simulink model "LEGO_HW"  (R2023a)
settings: Solver=ode3  StartTime=0.0  StopTime=inf  FixedStep=Ts  RelTol=1e-3
InitFcn:
  | lego_drive_openloop_InitData.mdl = get_param(bdroot,'Name');
  | lego_drive_openloop_InitData.cs = getActiveConfigSet(lego_drive_openloop_InitData.mdl);
values from neighbouring files (symbols this model uses):
  a_gc = 0.8    [run_LEGO_HW.m]
  a_gd = 0.999    [run_LEGO_HW.m]
  dot_phi_ref = -1.8    [run_LEGO_HW.m]
  dot_theta_ref = 7    [run_LEGO_HW.m]
  KDtheta = Kpp(3)    [run_LEGO_HW.m]
  KIpsi = Kpp(2)    [run_LEGO_HW.m]
  KItheta = Kpp(5)    [run_LEGO_HW.m]
  Kopenloop = -A2(2,2)/B2(2,1)    [run_LEGO_HW.m]
  KPphi = -6    [run_LEGO_HW.m]
  KPpsi = Kpp(4)    [run_LEGO_HW.m]
  KPtheta = Kpp(1)    [run_LEGO_HW.m]
  maxacc = 2    [run_LEGO_HW.m]
  R = 0.027    [run_LEGO_HW.m]
  thetamy = 2.8    [run_LEGO_HW.m]
  thres_yaw = -1    [run_LEGO_HW.m]
  Ts = 0.004    [run_LEGO_HW.m]
  W = 0.14    [run_LEGO_HW.m]
undefined symbols (not defined in the file or in its folder): DiscIntNeverNeededParam
libraries: legoev3lib x8, simulink x4, simulink_extras x3, shared_linuxserviceslib x1, simulink_need_slupdate x1
PreSaveFcn:
  | set_param(gcs, 'Location',[35 56 895 605])
CloseFcn:
  | clear lego_drive_openloop_InitData
settings Model: SimulationMode=external  ExtModeTrigDuration=2  Creator=The MathWorks, Inc.  LastModifiedBy=lab5
settings SolverCC: AlgebraicLoopSolver=TrustRegion  PositivePriorityOrder=on
settings DataIOCC: LimitDataPoints=on  SaveFormat=Array  SaveOutput=off  SignalLogging=off  DSMLogging=off  SaveTime=off  ReturnWorkspaceOutputs=off
settings OptimizationCC: ExpressionDepthLimit=2147483647  LifeSpan=Inf  MaxStackSize=64
settings DebuggingCC: UnderspecifiedInitializationDetection=Classic  MergeDetectMultiDrivingBlocksExec=none  InheritedTsInSrcMsg=none  ParameterPrecisionLossMsg=none  FcnCallInpInsideContextMsg=warning  UnconnectedInputMsg=warning  UnconnectedOutputMsg=warning  UnconnectedLineMsg=warning  AllowSymbolicDim=off  StateNameClashWarn=warning  SFUnexpectedBacktrackingDiag=warning  SFNoUnconditionalDefaultTransitionDiag=warning  SFExecutionAtInitializationDiag=none  ArithmeticOperatorsInVariantConditions=warning
settings HardwareCC: ProdBitPerPointer=32  ProdBitPerSizeT=32  ProdBitPerPtrDiffT=32  ProdLargestAtomicInteger=Long  ProdWordSize=32  ProdHWDeviceType=ARM Compatible->ARM 9  UseEmbeddedCoderFeatures=off  UseSimulinkCoderFeatures=off
settings ModelReferenceCC: UpdateModelReferenceTargets=Force  EnableRefExpFcnMdlSchedulingChecks=on  PropagateSignalLabelsOutOfModel=off
settings SFSimCC: SimUseLocalCustomCode=off  CustomCodeUndefinedFunction=UseInterfaceOnly
settings RTWCC: Description=Embedded Coder  SystemTargetFile=ert.tlc  HardwareBoard=LEGO MINDSTORMS EV3  TemplateMakefile=ert_default_tmf  GenerateReport=on  RTWVerbose=off  RTWUseLocalCustomCode=off  Toolchain=Sourcery G++ Lite v2009q3  LaunchReport=on  DLArmComputeVersion=19.05
settings CodeAppCC: ForceParamTrailComments=on  OperatorAnnotations=on  StateflowObjectComments=on  MATLABSourceComments=on
settings ERTTargetCC: MultiwordLength=2048  ERTCustomFileBanners=off  SupportContinuousTime=on  SupportNonInlinedSFcns=on  RemoveResetFunc=off  ModelStepFunctionPrototypeControlCompliant=off
settings ConfigComp: CovMetricSettings=dw  CovSaveCumulativeToWorkspaceVar=on  CovSaveSingleToWorkspaceVar=on  CovExternalEMLEnable=off  CovSFcnEnable=off

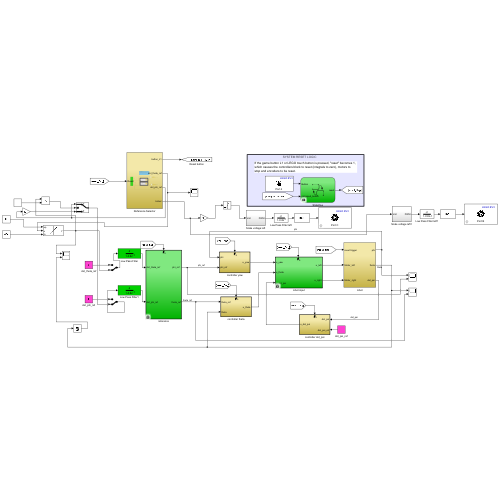
[thumbnail: Simulink's stored preview of the top-level diagram]
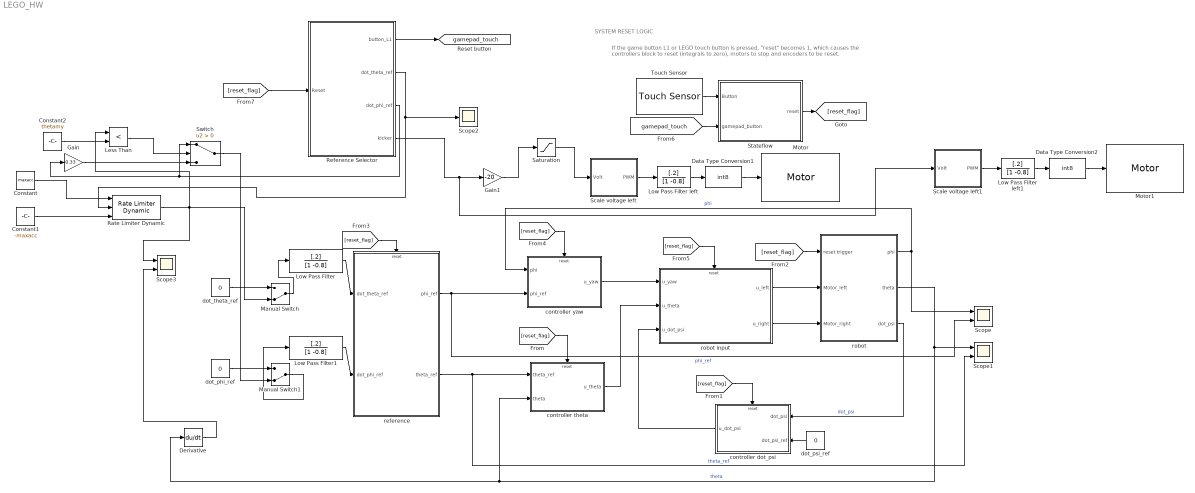
== system LEGO_HW ==
  note: If the game button L1 or LEGO touch button is pressed, "reset" becomes 1, which causes the controllers block to reset (integrals to zero), motors to stop and encoders to be reset.
  note: SYSTEM RESET LOGIC
  Constant : Constant  Value=maxacc
  Constant1 : Constant  Value=-maxacc
  Constant2 : Constant  Value=thetamy
  Data Type Conversion1 : DataTypeConversion  OutDataTypeStr=int8  SaturateOnIntegerOverflow=off  RndMeth=Floor
  Data Type Conversion2 : DataTypeConversion  OutDataTypeStr=int8  SaturateOnIntegerOverflow=off  RndMeth=Floor
  Derivative : Derivative
  Gain : Gain  Gain=0.33
  Gain1 : Gain  Gain=-20
  Less Than : RelationalOperator  Operator=<  OutDataTypeStr=boolean  RndMeth=Simplest  InputSameDT=off
  Low Pass Filter : DiscreteFilter  Numerator=[.2]  Denominator=[1 -0.8]  SampleTime=Ts
  Low Pass Filter left : DiscreteFilter  Numerator=[.2]  Denominator=[1 -0.8]
  Low Pass Filter left1 : DiscreteFilter  Numerator=[.2]  Denominator=[1 -0.8]
  Low Pass Filter1 : DiscreteFilter  Numerator=[.2]  Denominator=[1 -0.8]  SampleTime=Ts
  Manual Switch : ManualSwitch  CurrentSetting=0
  Manual Switch1 : ManualSwitch  CurrentSetting=0
  Motor : legoev3lib/Motor  sportNumber=C  sstopAction=Brake
  Motor1 : legoev3lib/Motor  sportNumber=B  sstopAction=Brake
  Rate Limiter Dynamic : simulink/Discontinuities/Rate Limiter Dynamic
  Reference Selector : Subsystem
  Saturation : Saturate  UpperLimit=2  LowerLimit=-20
  Scale voltage left : Subsystem
  Scale voltage left1 : Subsystem
  Scope : Scope  NumInputPorts=2
  Scope1 : Scope  NumInputPorts=2
  Scope2 : Scope
  Scope3 : Scope  NumInputPorts=2
  Stateflow : Stateflow chart  TreatAsAtomicUnit=on  SystemSampleTime=Ts
      settings: CopyFcn=|
      | % delete the link so that this is editable
      | set_param(gcb, 'LinkStatus', 'none');
  Switch : Switch  Criteria=u2 > Threshold  SaturateOnIntegerOverflow=off  InputSameDT=off
  Touch Sensor : legoev3lib/Touch Sensor  portNumber=4  sampleTime=Ts
  controller dot_psi : Subsystem
  controller theta : Subsystem
  controller yaw : Subsystem
  dot_phi_ref : Constant  Value=0
  dot_psi_ref : Constant  Value=0  VectorParams1D=off
  dot_theta_ref : Constant  Value=0
  reference : Subsystem
  robot : Subsystem  VariantControl=DoSim
  robot input : Subsystem
  tag scope: gamepad_touch=global
  wires:
  controller yaw/1(u_yaw) -> robot input/1(u_yaw)
  controller theta/1(u_theta) -> robot input/2(u_theta)
  controller dot_psi/1(u_dot_psi) -> robot input/3(u_dot_psi)
  reference/1("phi_ref  ") -> Scope/2, controller yaw/2(phi_ref)  "phi_ref"
  reference/2(theta_ref) -> Scope1/2, controller theta/1(theta_ref)  "theta_ref"
  dot_psi_ref/1 -> controller dot_psi/2(dot_psi_ref)
  robot/3(dot_psi) -> controller dot_psi/1(dot_psi)  "dot_psi"
  robot/2(theta) -> Derivative/1, controller theta/2(theta), Scope1/1  "theta"
  robot input/1(u_left) -> robot/2(Motor_left)
  robot input/2(u_right) -> robot/3(Motor_right)
  Stateflow/1(reset) -> [reset_flag]
  [reset_flag] -> controller theta/Reset
  [reset_flag] -> controller dot_psi/Reset
  [reset_flag] -> robot/1(reset trigger)
  [reset_flag] -> controller yaw/Reset
  [reset_flag] -> reference/Reset
  [reset_flag] -> robot input/Reset
  Touch Sensor/1 -> Stateflow/1(Button)
  robot/1(phi) -> controller yaw/1(phi), Scope/1  "phi"
  dot_theta_ref/1 -> Manual Switch/1
  dot_phi_ref/1 -> Manual Switch1/1
  [gamepad_touch] -> Stateflow/2(gamepad_button)
  Reference Selector/2(dot_theta_ref) -> Rate Limiter Dynamic/2, Scope2/1
  Reference Selector/4(kicker) -> Scale voltage left1/1(Volt), Gain1/1
  Reference Selector/1(button_L1) -> [gamepad_touch]
  [reset_flag] -> Reference Selector/1(Reset)
  Manual Switch/1 -> Low Pass Filter/1
  Low Pass Filter/1 -> reference/1(dot_theta_ref)
  Low Pass Filter1/1 -> reference/2(dot_phi_ref)
  Manual Switch1/1 -> Low Pass Filter1/1
  Constant/1 -> Rate Limiter Dynamic/1
  Constant1/1 -> Rate Limiter Dynamic/3
  Rate Limiter Dynamic/1 -> Less Than/1, Scope3/1, Manual Switch/2
  Derivative/1 -> Scope3/2
  Reference Selector/3(dot_phi_ref) -> Gain/1, Switch/1
  Switch/1 -> Manual Switch1/2
  Constant2/1 -> Less Than/2
  Less Than/1 -> Switch/2
  Gain/1 -> Switch/3
  Scale voltage left/1(PWM) -> Low Pass Filter left/1
  Low Pass Filter left/1 -> Data Type Conversion1/1
  Data Type Conversion1/1 -> Motor/1
  Gain1/1 -> Saturation/1
  Saturation/1 -> Scale voltage left/1(Volt)
  Scale voltage left1/1(PWM) -> Low Pass Filter left1/1
  Low Pass Filter left1/1 -> Data Type Conversion2/1
  Data Type Conversion2/1 -> Motor1/1

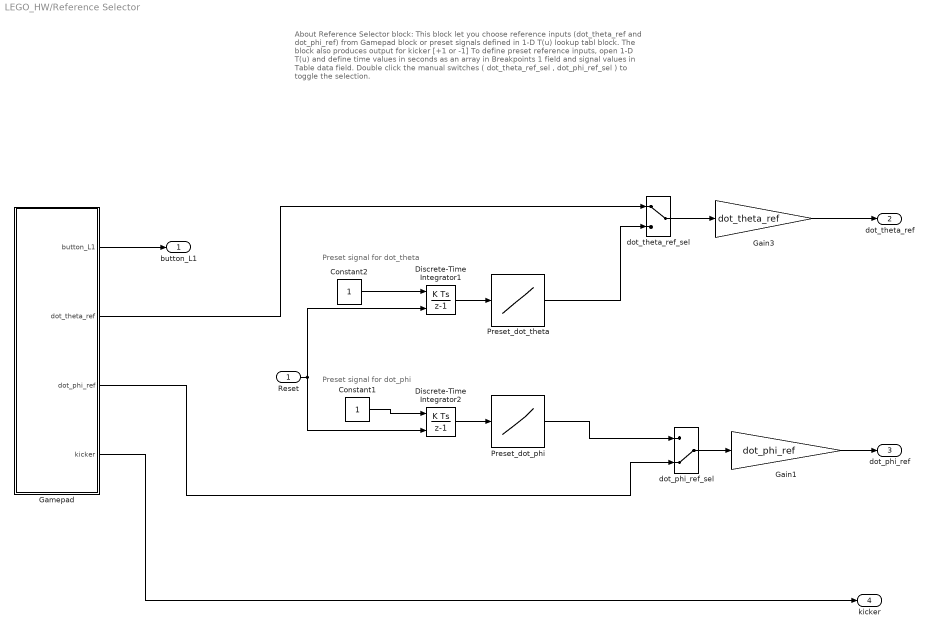
== system LEGO_HW/Reference Selector ==
  note: Preset signal for dot_theta
  note: About Reference Selector block:
      | This block let you choose reference inputs (dot_theta_ref and dot_phi_ref) from Gamepad block or preset signals defined in 1-D T(u) lookup tabl block. The block also produces output for kicker [+1 or -1]
      |
      | To define preset reference inputs, open 1-D T(u) and define time values in seconds as an array in Breakpoints 1 field and signal values in Table data field.
      |
      | Double click the manual switches ( dot_theta_ref_sel , dot_phi_ref_sel ) to toggle the selection.
  note: Preset signal for dot_phi
  Reset : Inport
  Constant1 : Constant
  Constant2 : Constant
  Discrete-Time Integrator1 : DiscreteIntegrator  ExternalReset=level  SampleTime=Ts  ICPrevOutput=DiscIntNeverNeededParam  ICPrevScaledInput=DiscIntNeverNeededParam
  Discrete-Time Integrator2 : DiscreteIntegrator  ExternalReset=level  SampleTime=Ts  ICPrevOutput=DiscIntNeverNeededParam  ICPrevScaledInput=DiscIntNeverNeededParam
  Gain1 : Gain  Gain=dot_phi_ref
  Gain3 : Gain  Gain=dot_theta_ref
  Gamepad : Subsystem
  Preset_dot_phi : Lookup_n-D  NumberOfTableDimensions=1  BreakpointsForDimension1=[0 1 2 3 4 5 6 9.1 10.8 11 12 12.1 12.2 13 14 15 16 17 18 19 20]  Table=[0;0;0;0;0;0;0;8;0;0;0;0;0;0;0;0;0;0;0;0;0]  InterpMethod=Flat  InternalRulePriority=Speed  RndMeth=Ceiling
  Preset_dot_theta : Lookup_n-D  NumberOfTableDimensions=1  BreakpointsForDimension1=[0;1;2;2.5;2.6;2.7;3.7;4.8;5.9;7;8;9;10;11;11.5;12.4;13;14;15;16;17;18;19;20;21;22]  Table=[0;0;0;0;0;0;0.5;1.5;2.5;2.7;2.5;1;0;0;0.5;1.3;2;2.3;2.5;2.1;1.5;0.5;0;0;0;0]  InterpMethod=Cubic spline  InternalRulePriority=Speed  RndMeth=Ceiling
  dot_phi_ref_sel : ManualSwitch  CurrentSetting=0
  dot_theta_ref_sel : ManualSwitch
  button_L1 : Outport
  dot_theta_ref : Outport  Port=2
  dot_phi_ref : Outport  Port=3
  kicker : Outport  Port=4
  wires:
  Discrete-Time Integrator1/1 -> Preset_dot_theta/1
  Gamepad/1(button_L1) -> button_L1/1
  Gamepad/2(dot_theta_ref) -> dot_theta_ref_sel/1
  Preset_dot_theta/1 -> dot_theta_ref_sel/2
  Gamepad/4(kicker) -> kicker/1
  dot_theta_ref_sel/1 -> Gain3/1
  dot_phi_ref_sel/1 -> Gain1/1
  Gain3/1 -> dot_theta_ref/1
  Discrete-Time Integrator2/1 -> Preset_dot_phi/1
  Reset/1 -> Discrete-Time Integrator2/2, Discrete-Time Integrator1/2
  Preset_dot_phi/1 -> dot_phi_ref_sel/1
  Gamepad/3(dot_phi_ref) -> dot_phi_ref_sel/2
  Gain1/1 -> dot_phi_ref/1
  Constant2/1 -> Discrete-Time Integrator1/1
  Constant1/1 -> Discrete-Time Integrator2/1

== system LEGO_HW/Scale voltage left ==
  Volt : Inport
  PWM --> Volts (for V_batt = 8000mV) : Gain  Gain=100/8.087
  Saturation : Saturate  UpperLimit=100  LowerLimit=-100
  PWM : Outport  VectorParamsAs1DForOutWhenUnconnected=off
  wires:
  PWM --> Volts (for V_batt = 8000mV)/1 -> Saturation/1
  Volt/1 -> PWM --> Volts (for V_batt = 8000mV)/1
  Saturation/1 -> PWM/1

== system LEGO_HW/Scale voltage left1 ==
  Volt : Inport
  PWM --> Volts (for V_batt = 8000mV) : Gain  Gain=100/8.087
  Saturation : Saturate  UpperLimit=100  LowerLimit=-100
  PWM : Outport  VectorParamsAs1DForOutWhenUnconnected=off
  wires:
  PWM --> Volts (for V_batt = 8000mV)/1 -> Saturation/1
  Volt/1 -> PWM --> Volts (for V_batt = 8000mV)/1
  Saturation/1 -> PWM/1

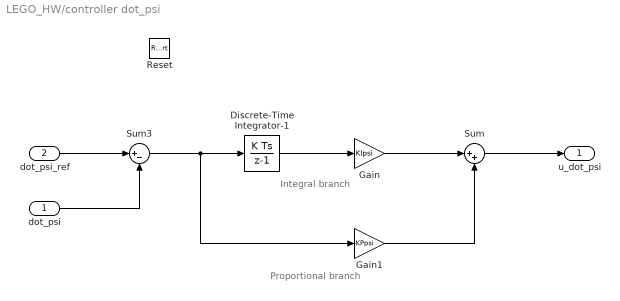
== system LEGO_HW/controller dot_psi ==
  note: Proportional branch
  note: Integral branch
  dot_psi : Inport
  dot_psi_ref : Inport  Port=2
  Reset : ResetPort  DisableCoverage=on
  Discrete-Time Integrator-1 : DiscreteIntegrator  SampleTime=Ts  ICPrevOutput=DiscIntNeverNeededParam  ICPrevScaledInput=DiscIntNeverNeededParam
  Gain : Gain  Gain=KIpsi
  Gain1 : Gain  Gain=KPpsi
  Sum : Sum  Inputs=|++  OutDataTypeStr=Inherit: Same as first input
  Sum3 : Sum  Inputs=|+-  OutDataTypeStr=Inherit: Same as first input
  u_dot_psi : Outport  VectorParamsAs1DForOutWhenUnconnected=off
  wires:
  dot_psi/1 -> Sum3/2
  dot_psi_ref/1 -> Sum3/1
  Discrete-Time Integrator-1/1 -> Gain/1
  Sum3/1 -> Gain1/1, Discrete-Time Integrator-1/1
  Sum/1 -> u_dot_psi/1
  Gain1/1 -> Sum/2
  Gain/1 -> Sum/1

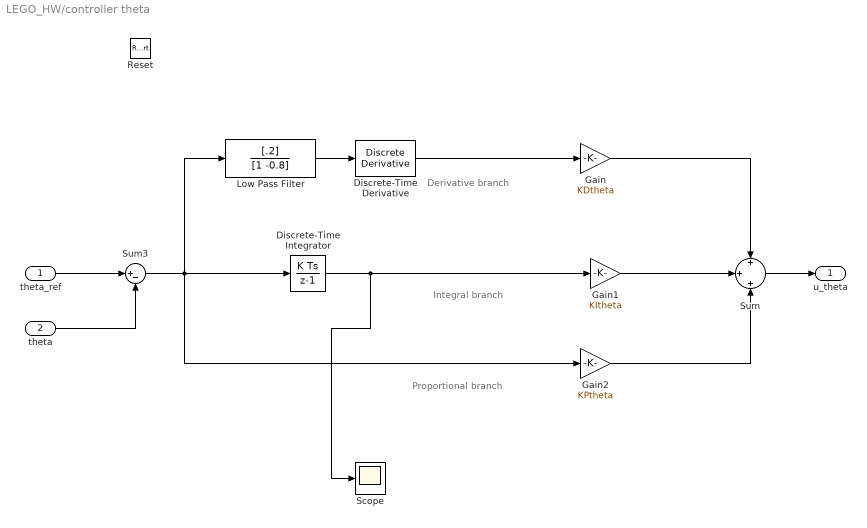
== system LEGO_HW/controller theta ==
  note: Proportional branch
  note: Integral branch
  note: Derivative branch
  theta_ref : Inport
  theta : Inport  Port=2
  Reset : ResetPort  DisableCoverage=on
  Discrete-Time Derivative : simulink/Discrete/Discrete Derivative  gainval=1.0  ICPrevScaledInput=0.0  OutMin=[]  OutMax=[]  OutDataType=fixdt(1, 16)  OutScaling=2^-10  DoSatur=off
  Discrete-Time Integrator : DiscreteIntegrator  SampleTime=Ts  ICPrevOutput=DiscIntNeverNeededParam  ICPrevScaledInput=DiscIntNeverNeededParam
  Gain : Gain  Gain=KDtheta
  Gain1 : Gain  Gain=KItheta
  Gain2 : Gain  Gain=KPtheta
  Low Pass Filter : DiscreteFilter  Numerator=[.2]  Denominator=[1 -0.8]  SampleTime=Ts
  Scope : Scope
  Sum : Sum  Inputs=+|+|+  OutDataTypeStr=Inherit: Same as first input
  Sum3 : Sum  Inputs=|+-  OutDataTypeStr=Inherit: Same as first input
  u_theta : Outport  VectorParamsAs1DForOutWhenUnconnected=off
  wires:
  theta/1 -> Sum3/2
  theta_ref/1 -> Sum3/1
  Discrete-Time Integrator/1 -> Scope/1, Gain1/1
  Discrete-Time Derivative/1 -> Gain/1
  Sum3/1 -> Gain2/1, Discrete-Time Integrator/1, Low Pass Filter/1
  Sum/1 -> u_theta/1
  Gain2/1 -> Sum/3
  Gain1/1 -> Sum/2
  Gain/1 -> Sum/1
  Low Pass Filter/1 -> Discrete-Time Derivative/1

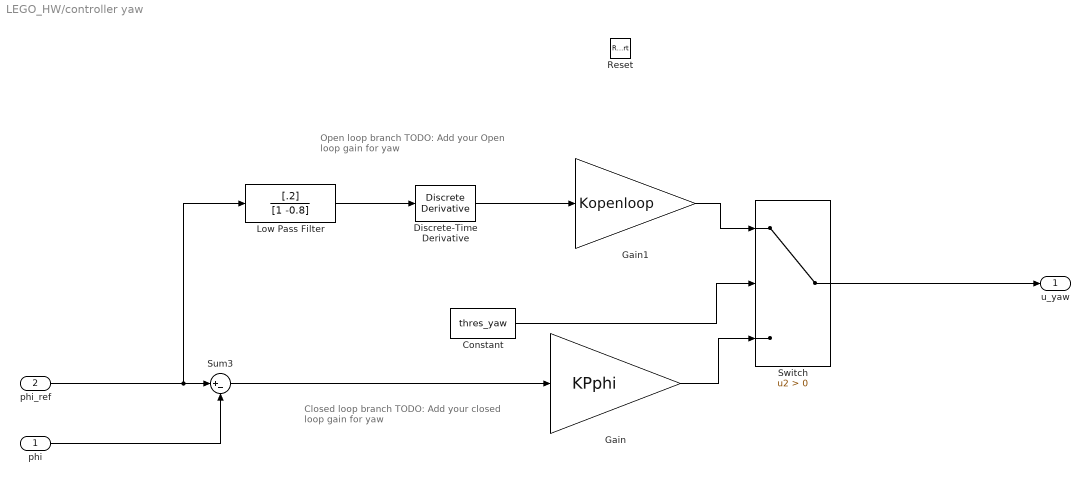
== system LEGO_HW/controller yaw ==
  note: Closed loop branch
      | TODO: Add your closed loop gain for yaw
  note: Open loop branch
      | TODO: Add your Open loop gain for yaw
  phi : Inport
  phi_ref : Inport  Port=2
  Reset : ResetPort  DisableCoverage=on
  Constant : Constant  Value=thres_yaw
  Discrete-Time Derivative : simulink/Discrete/Discrete Derivative  gainval=1.0  ICPrevScaledInput=0.0  OutMin=[]  OutMax=[]  OutDataType=fixdt(1, 16)  OutScaling=2^-10  DoSatur=off
  Gain : Gain  Gain=KPphi
  Gain1 : Gain  Gain=Kopenloop
  Low Pass Filter : DiscreteFilter  Numerator=[.2]  Denominator=[1 -0.8]  SampleTime=Ts
  Sum3 : Sum  Inputs=|+-
  Switch : Switch  Criteria=u2 > Threshold  SaturateOnIntegerOverflow=off  InputSameDT=off
  u_yaw : Outport  VectorParamsAs1DForOutWhenUnconnected=off
  wires:
  phi/1 -> Sum3/2
  phi_ref/1 -> Low Pass Filter/1, Sum3/1
  Sum3/1 -> Gain/1
  Discrete-Time Derivative/1 -> Gain1/1
  Constant/1 -> Switch/2
  Low Pass Filter/1 -> Discrete-Time Derivative/1
  Gain1/1 -> Switch/1
  Switch/1 -> u_yaw/1
  Gain/1 -> Switch/3

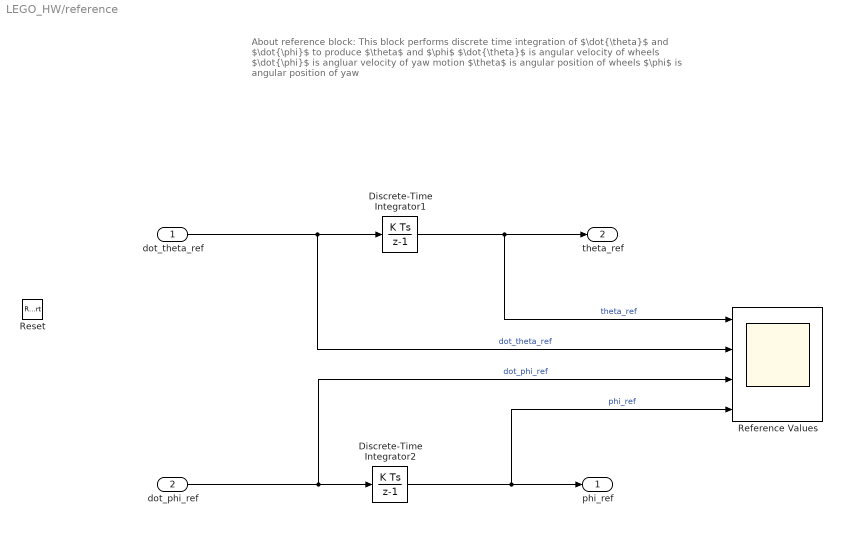
== system LEGO_HW/reference ==
  note: About reference block:
      | This block performs discrete time integration of $\dot{\theta}$ and $\dot{\phi}$ to produce $\theta$ and $\phi$
      | $\dot{\theta}$ is angular velocity of wheels
      | $\dot{\phi}$ is angluar velocity of yaw motion
      | $\theta$ is angular position of wheels
      | $\phi$ is angular position of yaw
  dot_theta_ref : Inport
  dot_phi_ref : Inport  Port=2
  Reset : ResetPort  DisableCoverage=on
  Discrete-Time Integrator1 : DiscreteIntegrator  SampleTime=Ts  ICPrevOutput=DiscIntNeverNeededParam  ICPrevScaledInput=DiscIntNeverNeededParam
  Discrete-Time Integrator2 : DiscreteIntegrator  SampleTime=Ts  ICPrevOutput=DiscIntNeverNeededParam  ICPrevScaledInput=DiscIntNeverNeededParam
  Reference Values : Scope  NumInputPorts=4
  "phi_ref  " : Outport  VectorParamsAs1DForOutWhenUnconnected=off
  theta_ref : Outport  Port=2  VectorParamsAs1DForOutWhenUnconnected=off
  wires:
  dot_phi_ref/1 -> Reference Values/3, Discrete-Time Integrator2/1  "dot_phi_ref"
  Discrete-Time Integrator2/1 -> Reference Values/4, "phi_ref  "/1  "phi_ref"
  Discrete-Time Integrator1/1 -> Reference Values/1, theta_ref/1  "theta_ref"
  dot_theta_ref/1 -> Reference Values/2, Discrete-Time Integrator1/1  "dot_theta_ref"

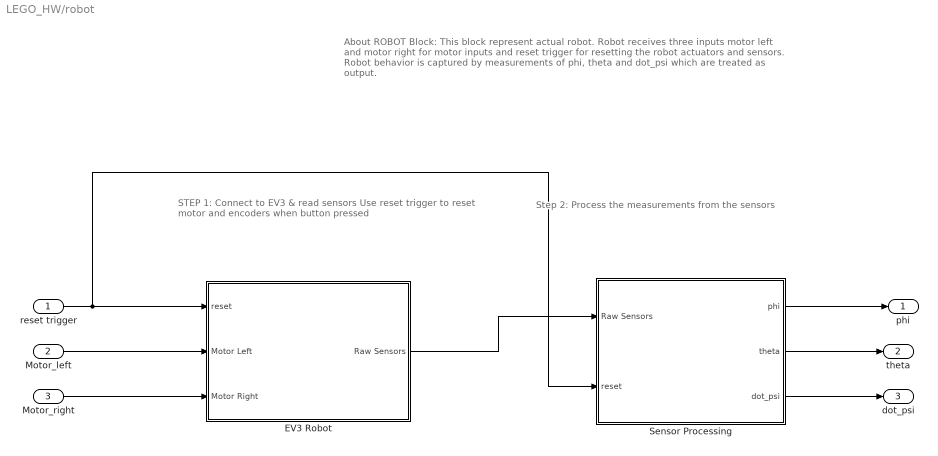
== system LEGO_HW/robot ==
  note: STEP 1: Connect to EV3 & read sensors
      |
      | Use reset trigger to reset motor and encoders
      | when button pressed
  note: Step 2: Process the measurements from the sensors
  note: About ROBOT Block:
      |
      | This block represent actual robot. Robot receives three inputs motor left and motor right for motor inputs and reset trigger for resetting the robot actuators and sensors.
      | Robot behavior is captured by measurements of phi, theta and dot_psi which are treated as output.
  reset trigger : Inport
  Motor_left : Inport  Port=2
  Motor_right : Inport  Port=3
  EV3 Robot : Subsystem
  Sensor Processing : Subsystem  TreatAsAtomicUnit=on
  phi : Outport  VectorParamsAs1DForOutWhenUnconnected=off
  theta : Outport  Port=2  VectorParamsAs1DForOutWhenUnconnected=off
  dot_psi : Outport  Port=3  VectorParamsAs1DForOutWhenUnconnected=off
  wires:
  Sensor Processing/2(theta) -> theta/1
  Sensor Processing/3(dot_psi) -> dot_psi/1
  Sensor Processing/1(phi) -> phi/1
  EV3 Robot/1(Raw Sensors) -> Sensor Processing/1(Raw Sensors)
  Motor_right/1 -> EV3 Robot/3(Motor Right)
  Motor_left/1 -> EV3 Robot/2(Motor Left)
  reset trigger/1 -> Sensor Processing/2(reset), EV3 Robot/1(reset)

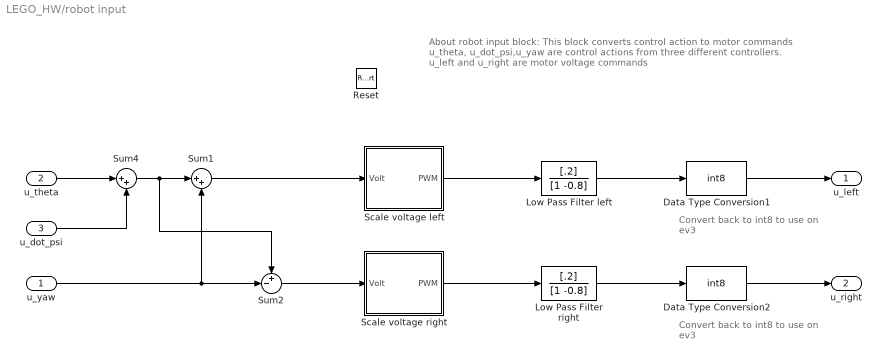
== system LEGO_HW/robot input ==
  note: About robot input block:
      | This block converts control action to motor commands
      | u_theta, u_dot_psi,u_yaw are control actions from three different controllers.
      | u_left and u_right are motor voltage commands
  note: Convert back to int8 to use on ev3
  note: Convert back to int8 to use on ev3
  u_yaw : Inport
  u_theta : Inport  Port=2
  u_dot_psi : Inport  Port=3
  Reset : ResetPort  DisableCoverage=on
  Data Type Conversion1 : DataTypeConversion  OutDataTypeStr=int8  SaturateOnIntegerOverflow=off  RndMeth=Floor
  Data Type Conversion2 : DataTypeConversion  OutDataTypeStr=int8  SaturateOnIntegerOverflow=off  RndMeth=Floor
  Low Pass Filter left : DiscreteFilter  Numerator=[.2]  Denominator=[1 -0.8]
  Low Pass Filter right : DiscreteFilter  Numerator=[.2]  Denominator=[1 -0.8]
  Scale voltage left : Subsystem
  Scale voltage right : Subsystem
  Sum1 : Sum  Inputs=|++
  Sum2 : Sum  Inputs=+-|
  Sum4 : Sum  Inputs=|++
  u_left : Outport  VectorParamsAs1DForOutWhenUnconnected=off
  u_right : Outport  Port=2  VectorParamsAs1DForOutWhenUnconnected=off
  wires:
  Scale voltage left/1(PWM) -> Low Pass Filter left/1
  Low Pass Filter left/1 -> Data Type Conversion1/1
  u_theta/1 -> Sum4/1
  u_dot_psi/1 -> Sum4/2
  u_yaw/1 -> Sum2/2, Sum1/2
  Sum4/1 -> Sum2/1, Sum1/1
  Sum2/1 -> Scale voltage right/1(Volt)
  Sum1/1 -> Scale voltage left/1(Volt)
  Scale voltage right/1(PWM) -> Low Pass Filter right/1
  Low Pass Filter right/1 -> Data Type Conversion2/1
  Data Type Conversion1/1 -> u_left/1
  Data Type Conversion2/1 -> u_right/1

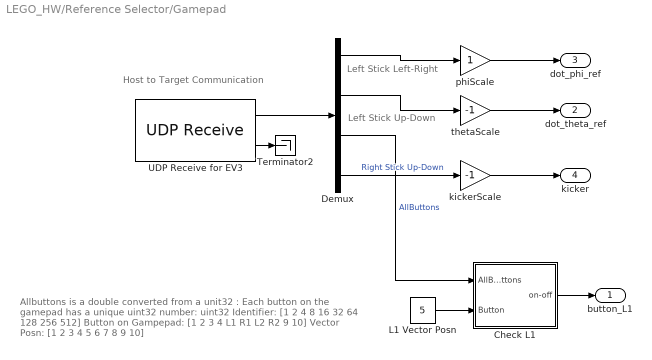
== system LEGO_HW/Reference Selector/Gamepad ==
  note: Left Stick Left-Right
  note: Host to Target Communication
  note: Left Stick Up-Down
  note: Allbuttons is a double converted from a unit32 :
      | Each button on the gamepad has a unique uint32 number:
      | uint32 Identifier: [1 2 4 8 16 32 64 128 256 512]
      | Button on Gampepad: [1 2 3 4 L1 R1 L2 R2 9 10]
      | Vector Posn: [1 2 3 4 5 6 7 8 9 10]
  Check L1 : Subsystem
  Demux : Demux
  L1 Vector Posn : Constant  Value=5
  Terminator2 : Terminator
  UDP Receive for EV3 : shared_linuxserviceslib/UDP Receive  localURL='0.0.0.0'  localPort=3  remoteURL='0.0.0.0'  remotePort=-1  recvBufferSize=8192  signalDatatype=double  dims=4  isVarSize=off  showBlockingTime=off  blockingTime=0  sampletime=Ts  blockPlatform=LEGO EV3
  kickerScale : Gain  Gain=-1
  phiScale : Gain
  thetaScale : Gain  Gain=-1
  button_L1 : Outport  VectorParamsAs1DForOutWhenUnconnected=off
  dot_theta_ref : Outport  Port=2  VectorParamsAs1DForOutWhenUnconnected=off
  dot_phi_ref : Outport  Port=3  VectorParamsAs1DForOutWhenUnconnected=off
  kicker : Outport  Port=4  VectorParamsAs1DForOutWhenUnconnected=off
  wires:
  Demux/1 -> phiScale/1
  UDP Receive for EV3/2 -> Terminator2/1
  UDP Receive for EV3/1 -> Demux/1
  Demux/2 -> thetaScale/1
  Demux/3 -> Check L1/1("AllButtons ")  "AllButtons"
  thetaScale/1 -> dot_theta_ref/1
  phiScale/1 -> dot_phi_ref/1
  L1 Vector Posn/1 -> Check L1/2(Button)
  Check L1/1(on-off) -> button_L1/1
  kickerScale/1 -> kicker/1
  Demux/4 -> kickerScale/1  "Right Stick Up-Down"

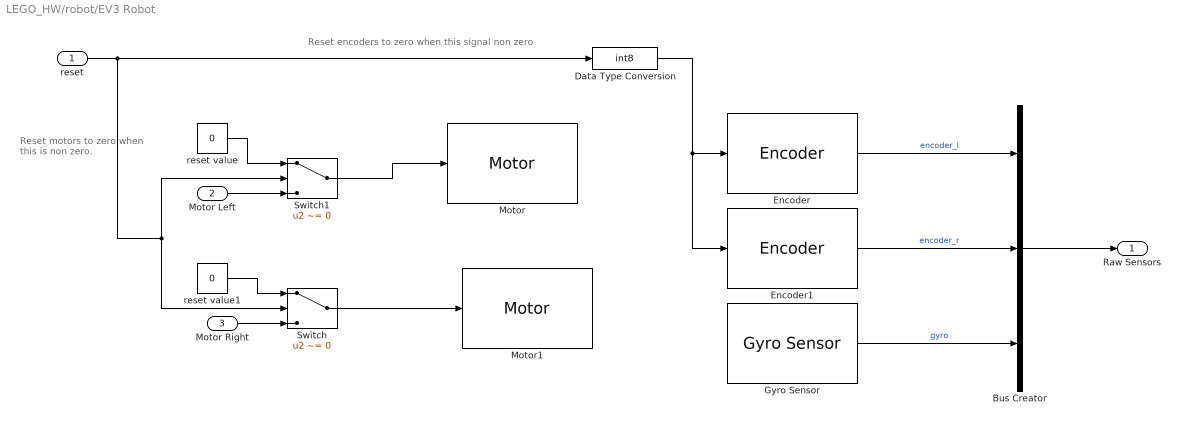
== system LEGO_HW/robot/EV3 Robot ==
  note: Reset motors to zero when this is non zero.
  note: Reset encoders to zero when this signal non zero
  reset : Inport
  Motor Left : Inport  Port=2
  Motor Right : Inport  Port=3
  Bus Creator : BusCreator  Inputs=3
  Data Type Conversion : DataTypeConversion  OutDataTypeStr=int8  SaturateOnIntegerOverflow=off  RndMeth=Floor
  Encoder : legoev3lib/Encoder  portNumber=D  opMode=Reset by external signal  sampleTime=Ts
  Encoder1 : legoev3lib/Encoder  portNumber=A  opMode=Reset by external signal  sampleTime=Ts
  Gyro Sensor : legoev3lib/Gyro Sensor  portNumber=3  sampleTime=Ts
  Motor : legoev3lib/Motor  sportNumber=D  sstopAction=Brake
  Motor1 : legoev3lib/Motor  sportNumber=A  sstopAction=Brake
  Switch : Switch  Criteria=u2 ~= 0  SaturateOnIntegerOverflow=off  InputSameDT=off
  Switch1 : Switch  Criteria=u2 ~= 0  Threshold=1  SaturateOnIntegerOverflow=off  InputSameDT=off
  reset value : Constant  Value=0
  reset value1 : Constant  Value=0
  Raw Sensors : Outport  VectorParamsAs1DForOutWhenUnconnected=off
  wires:
  Bus Creator/1 -> Raw Sensors/1
  reset/1 -> Switch1/2, Switch/2, Data Type Conversion/1
  Switch1/1 -> Motor/1
  Switch/1 -> Motor1/1
  Motor Right/1 -> Switch/3
  Motor Left/1 -> Switch1/3
  reset value/1 -> Switch1/1
  reset value1/1 -> Switch/1
  Encoder/1 -> Bus Creator/1  "encoder_l"
  Encoder1/1 -> Bus Creator/2  "encoder_r"
  Gyro Sensor/1 -> Bus Creator/3  "gyro"
  Data Type Conversion/1 -> Encoder1/1, Encoder/1

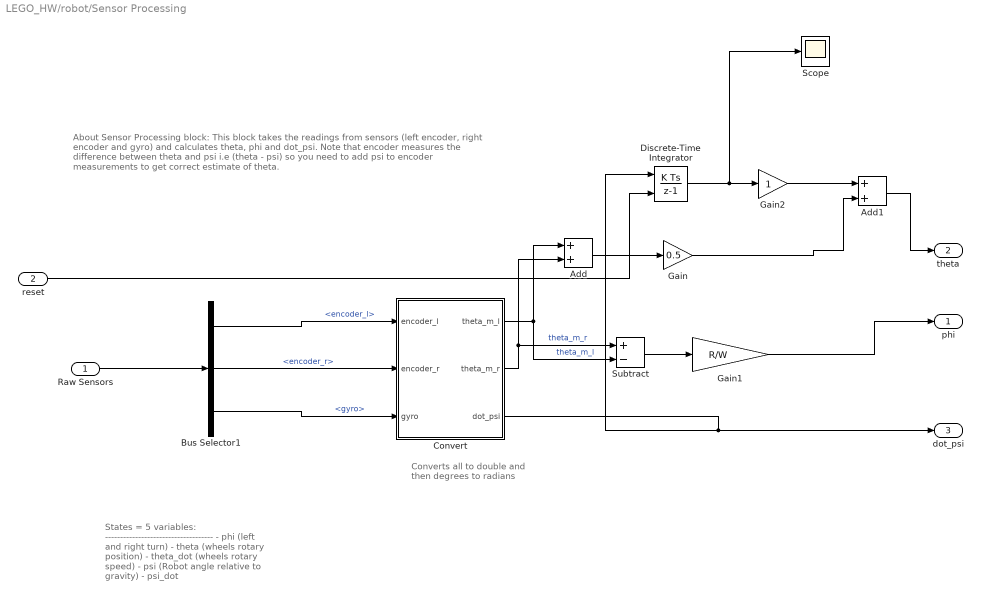
== system LEGO_HW/robot/Sensor Processing ==
  note: Converts all to double and then degrees to radians
  note: States = 5 variables:
      | ------------------------------------
      | - phi (left and right turn)
      | - theta (wheels rotary position)
      | - theta_dot (wheels rotary speed)
      | - psi (Robot angle relative to gravity)
      | - psi_dot
  note: About Sensor Processing block:
      | This block takes the readings from sensors (left encoder, right encoder and gyro) and calculates theta, phi and dot_psi.
      |
      | Note that encoder measures the difference between theta and psi i.e  (theta - psi) so you need to add psi to encoder measurements to get correct estimate of theta.
  Raw Sensors : Inport
  reset : Inport  Port=2
  Add : Sum
  Add1 : Sum
  Bus Selector1 : BusSelector  OutputSignals=encoder_l,encoder_r,gyro
  Convert : Subsystem
  Discrete-Time Integrator : DiscreteIntegrator  ExternalReset=rising  SampleTime=Ts  ICPrevOutput=DiscIntNeverNeededParam  ICPrevScaledInput=DiscIntNeverNeededParam
  Gain : Gain  Gain=0.5
  Gain1 : Gain  Gain=R/W
  Gain2 : Gain
  Scope : Scope
  Subtract : Sum  Inputs=+-
  phi : Outport  VectorParamsAs1DForOutWhenUnconnected=off
  theta : Outport  Port=2  VectorParamsAs1DForOutWhenUnconnected=off
  dot_psi : Outport  Port=3  VectorParamsAs1DForOutWhenUnconnected=off
  wires:
  Raw Sensors/1 -> Bus Selector1/1
  Bus Selector1/1 -> Convert/1(encoder_l)  "<encoder_l>"
  Bus Selector1/2 -> Convert/2(encoder_r)  "<encoder_r>"
  Bus Selector1/3 -> Convert/3(gyro)  "<gyro>"
  Convert/3(dot_psi) -> dot_psi/1, Discrete-Time Integrator/1
  Add/1 -> Gain/1
  Convert/1(theta_m_l) -> Add/1, Subtract/2  "theta_m_l"
  Convert/2(theta_m_r) -> Subtract/1, Add/2  "theta_m_r"
  Gain/1 -> Add1/2
  Subtract/1 -> Gain1/1
  Gain1/1 -> phi/1
  Add1/1 -> theta/1
  Discrete-Time Integrator/1 -> Scope/1, Gain2/1
  Gain2/1 -> Add1/1
  reset/1 -> Discrete-Time Integrator/2

== system LEGO_HW/robot input/Scale voltage left ==
  Volt : Inport
  PWM --> Volts (for V_batt = 8000mV) : Gain  Gain=100/8.087
  Saturation : Saturate  UpperLimit=100  LowerLimit=-100
  PWM : Outport  VectorParamsAs1DForOutWhenUnconnected=off
  wires:
  PWM --> Volts (for V_batt = 8000mV)/1 -> Saturation/1
  Volt/1 -> PWM --> Volts (for V_batt = 8000mV)/1
  Saturation/1 -> PWM/1

== system LEGO_HW/robot input/Scale voltage right ==
  Volt : Inport
  PWM --> Volts (for V_batt = 8000mV) : Gain  Gain=100/8.087
  Saturation : Saturate  UpperLimit=100  LowerLimit=-100
  PWM : Outport  VectorParamsAs1DForOutWhenUnconnected=off
  wires:
  PWM --> Volts (for V_batt = 8000mV)/1 -> Saturation/1
  Volt/1 -> PWM --> Volts (for V_batt = 8000mV)/1
  Saturation/1 -> PWM/1

== system LEGO_HW/Reference Selector/Gamepad/Check L1 ==
  note: AllButtons is now 1D vector with 10 elements (binary 0/1 if the button has been pressed)
  note: Block to Convert gamepad button output (unit32) to a vector of 1s and 0s, and checks for single button being pressed
  note: Convert the double (which was an unit32) to a binary output
  note: The input of this block is the original output from the Gampepad:
      | A unint32 number corresponding to which buttons are pressed:
      | Each button has a unique uint32 number:
      | uint32 Identifier: [1 2 4 8 16 32 64 128 256 512]
      | Button on Gampepad: [1 2 3 4 L1 R1 L2 R2 9 10]
      | Vector Posn: [1 2 3 4 5 6 7 8 9 10]
  note: Grab the element, corresponding to if button X has been pressed where X is external input 2.
      | e.g. if Button is 5 this block checks for L1 being pressed
  "AllButtons " : Inport
  Button : Inport  Port=2
  Display1 : Display
  Integer to Bit Converter : simulink/Logic and Bit Operations/Integer to Bit Converter  nbits=10  signedInputValues=Unsigned  bitOrder=LSB first  outDtype=Inherit via internal rule
      settings: LibrarySourceBlock=|
      | commutil2/Integer to Bit
      | Converter
  Selector : Selector  InputPortWidth=10  IndexOptions=Index vector (port)  Indices=[1]  OutputSizes=1
  on-off : Outport  VectorParamsAs1DForOutWhenUnconnected=off
  wires:
  "AllButtons "/1 -> Integer to Bit Converter/1
  Integer to Bit Converter/1 -> Selector/1, Display1/1
  Selector/1 -> on-off/1
  Button/1 -> Selector/2

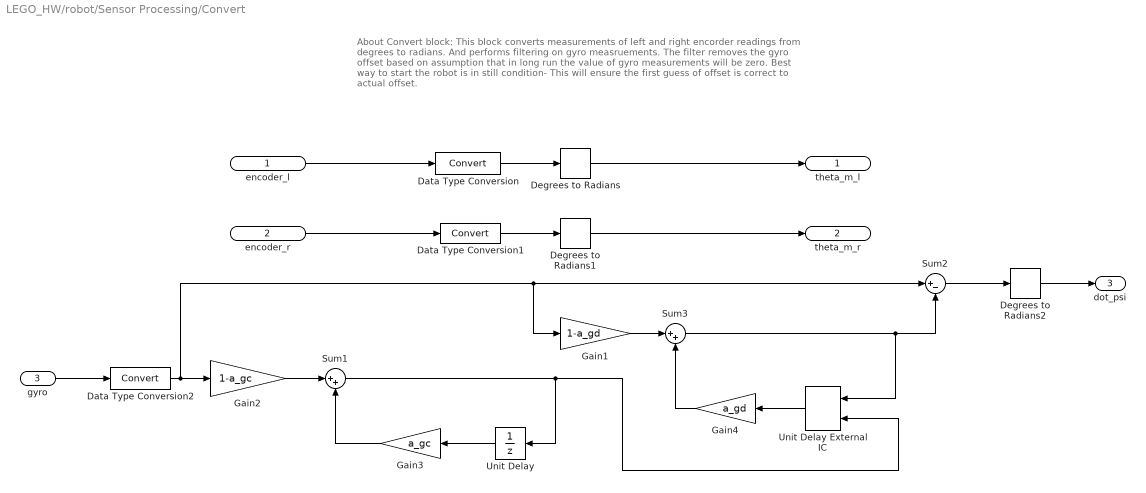
== system LEGO_HW/robot/Sensor Processing/Convert ==
  note: About Convert block:
      | This block converts measurements of left and right encorder readings from degrees to radians. And performs filtering on gyro measruements.
      | The filter removes the gyro offset based on assumption that in long run the value of gyro measurements will be zero.
      | Best way to start the robot is in still condition- This will ensure the first guess of offset is correct to actual offset.
  encoder_l : Inport
  encoder_r : Inport  Port=2
  gyro : Inport  Port=3
  Data Type Conversion : DataTypeConversion  SaturateOnIntegerOverflow=off  RndMeth=Floor
  Data Type Conversion1 : DataTypeConversion  SaturateOnIntegerOverflow=off  RndMeth=Floor
  Data Type Conversion2 : DataTypeConversion  SaturateOnIntegerOverflow=off  RndMeth=Floor
  Degrees to Radians : simulink_extras/Transformations/Degrees to Radians
  Degrees to Radians1 : simulink_extras/Transformations/Degrees to Radians
  Degrees to Radians2 : simulink_extras/Transformations/Degrees to Radians
  Gain1 : Gain  Gain=1-a_gd  OutDataTypeStr=Inherit: Same as input  ParamDataTypeStr=Inherit: Same as input
  Gain2 : Gain  Gain=1-a_gc  OutDataTypeStr=Inherit: Same as input  ParamDataTypeStr=Inherit: Same as input
  Gain3 : Gain  Gain=a_gc  OutDataTypeStr=Inherit: Same as input  ParamDataTypeStr=Inherit: Same as input
  Gain4 : Gain  Gain=a_gd  OutDataTypeStr=Inherit: Same as input  ParamDataTypeStr=Inherit: Same as input
  Sum1 : Sum  Inputs=|++  OutDataTypeStr=Inherit: Same as first input
  Sum2 : Sum  Inputs=|+-  OutDataTypeStr=Inherit: Same as first input
  Sum3 : Sum  Inputs=|++  OutDataTypeStr=Inherit: Same as first input
  Unit Delay : UnitDelay  SampleTime=-1  HasFrameUpgradeWarning=on
  Unit Delay External IC : simulink_need_slupdate/Unit Delay External IC  tsamp=-1
  theta_m_l : Outport  VectorParamsAs1DForOutWhenUnconnected=off
  theta_m_r : Outport  Port=2  VectorParamsAs1DForOutWhenUnconnected=off
  dot_psi : Outport  Port=3  VectorParamsAs1DForOutWhenUnconnected=off
  wires:
  encoder_l/1 -> Data Type Conversion/1
  Data Type Conversion/1 -> Degrees to Radians/1
  encoder_r/1 -> Data Type Conversion1/1
  Data Type Conversion1/1 -> Degrees to Radians1/1
  Degrees to Radians/1 -> theta_m_l/1
  Degrees to Radians1/1 -> theta_m_r/1
  Degrees to Radians2/1 -> dot_psi/1
  Gain3/1 -> Sum1/2
  Unit Delay/1 -> Gain3/1
  Gain2/1 -> Sum1/1
  gyro/1 -> Data Type Conversion2/1
  Data Type Conversion2/1 -> Gain1/1, Sum2/1, Gain2/1
  Sum2/1 -> Degrees to Radians2/1
  Sum3/1 -> Sum2/2, Unit Delay External IC/1
  Sum1/1 -> Unit Delay External IC/2, Unit Delay/1
  Gain1/1 -> Sum3/1
  Unit Delay External IC/1 -> Gain4/1
  Gain4/1 -> Sum3/2

== stateflow chart LEGO_HW/Stateflow ==
  state STARTUP_RESET
    entry: reset=1;
  note: Start in Reset Mode
      | Motors are stopped
      | Encoder reads zero
  state READY
    entry: reset=1
  note: If the button on the EV3
      | OR
      | the button on the Gamepad
      | has been pressed then RESET
  note: If the button on the EV3
      | OR
      | the button on the Gamepad
      | has been pressed then READY
  state READY1
    entry: reset=0
  state READY2
    entry: reset=1
  state RUNMODE
    entry: reset=0
  note: MAIN RUN MODE
  note: In RESET mode the integrals are reset to zero and the motors are stopped
  state RESET
    entry: reset=1
  note: Once neither the button on the EV3 or the button on the Gampad are presssed, wait 0.05 seconds after last release and start balancing again.
  state RESET1FINAL
    entry: reset=1
  (default) -> STARTUP_RESET
  RESET1FINAL -> STARTUP_RESET : after(0.05,sec)
  STARTUP_RESET -> READY : [(Button==1)||(gamepad_button==1)==1]
  READY -> READY1 : [(Button==0)&&(gamepad_button==0)]
  READY1 -> READY2 : after(0.05,sec)
  READY2 -> RUNMODE : after(0.05,sec)
  RUNMODE -> RESET : [Button==1 || gamepad_button==1]
  RESET -> RESET1FINAL : [(Button==0)&&(gamepad_button==0)]
  data: Button input; reset output double; gamepad_button input double
